simulink model "BaseMotorControl"  (R2025a)
settings: Solver=FixedStepAuto  StartTime=0.0  StopTime=T_total  FixedStep=25e-6  RelTol=1e-3
StartFcn:
  | learning.simulink.modelCallbacks.startFunction(gcs)
StopFcn:
  | learning.simulink.modelCallbacks.stopFunction(gcs);
model workspace (MAT data in the model file):
  courseObject.course = 'otslimc'
  courseObject.chapter = 5
  courseObject.lesson = 1
  courseObject.section = 3
  courseObject.task = 1
  t_ans = [0 2.5e-05 5e-05 7.5e-05 0.0001 0.000125 0.00015 0.000175 0.0002 0.000225 0.00025 0.000275 ... (2001 elements, 2001x1)]
  y_ans = [0 0 0.052825565971 0.155642198422 0.305764234901 0.500647055712 0.737879693209 1.01517782556 1.33037713629 1.68142702156 2.06638462754 2.48340920133 ... (2001 elements, 2001x1)]
values from neighbouring files (symbols this model uses):
  pmsm =     [pmsm_values.mat]    (also in sample_time.mat)
  Ts = 2.5000e-05    (= 2.5e-05)    [System_Parameters.m]    (also in pmsm_values.mat; sample_time.mat)
libraries: mcbcontrollergainlib x4, mcbfoclib x2, mcbpositiondecoderlib x2, mcbplantlib x2, autolibpmsminterior x2, slpidlib x2
(part 1 of 2)
CloseFcn:
  | learning.simulink.cleanupOnlineTraining;learning.simulink.Application.getInstance().dduxLogMatlabEvent("ModelClosed")
Description:
  | TrainingCourseModel
settings Model: Creator=mac  LastModifiedBy=mac
settings DataIOCC: SaveTime=off
settings DebuggingCC: ParamSuppressDoubleToSinglePrecisionLossMsg=on
settings RTWCC: GPUComputeCapability=3.5

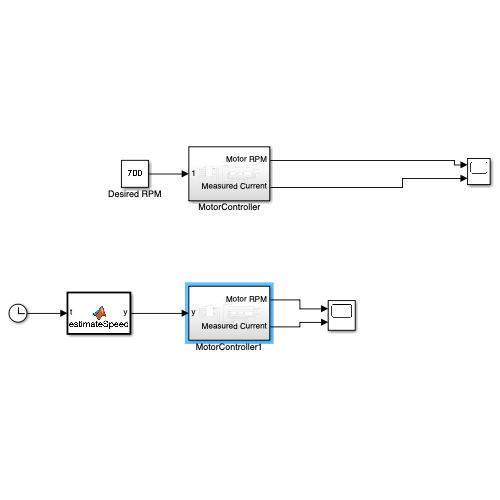
[thumbnail: Simulink's stored preview of the top-level diagram]
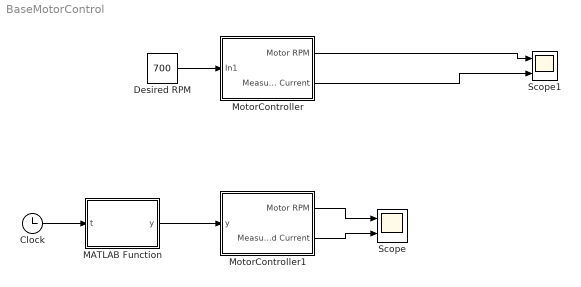
== system BaseMotorControl ==
  Clock : Clock
  Desired RPM : Constant  Value=700
  MATLAB Function : MATLAB Function  TreatAsAtomicUnit=on
  MotorController : Subsystem
  MotorController1 : Subsystem
  Scope : Scope  NumInputPorts=2
      settings: ActiveDisplayYMinimum=-312.679673846435  ActiveDisplayYMaximum=810.75563817244858
  Scope1 : Scope  NumInputPorts=2
      settings: ActiveDisplayYMinimum=-91.459957244733559  ActiveDisplayYMaximum=823.13961520260216
  wires:
  Desired RPM/1 -> MotorController/1(In1)
  Clock/1 -> MATLAB Function/1(t)
  MATLAB Function/1(y) -> MotorController1/1(y)
  MotorController/1(Motor RPM) -> Scope1/1
  MotorController/2(Measured Current) -> Scope1/2
  MotorController1/1(Motor RPM) -> Scope/1
  MotorController1/2(Measured Current) -> Scope/2
